simulink model "blockdemo_accumulationchaining"  (Simulink 7.6)
settings: Solver=ode45  StartTime=0.0  StopTime=10.0  RelTol=1e-3
InitFcn:
  | %% DSPBuilder Start
  | alt_dspbuilder_update_model(bdroot)
  | %% DSPBuilder End
libraries: allblocks_alteradspbuilder2 x14, simulink x2
settings Model: Creator=akarapet  LastModifiedBy=akarapet

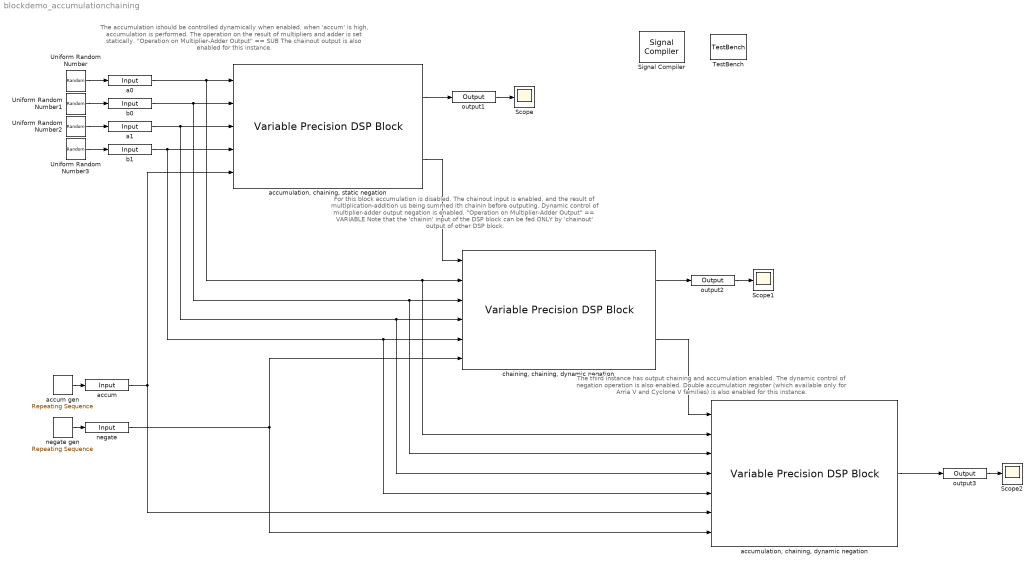
== system blockdemo_accumulationchaining ==
  note: The accumulation ishould be controlled dynamically when enabled.
      | when 'accum' is high, accumulation is performed.
      | The operation on the result of multipliers and adder is set statically.
      | "Operation on Multiplier-Adder Output" == SUB
      | The chainout output is also enabled for this instance.
  note: For this block accumulation is disabled.
      | The chainout input is enabled, and the result of multiplication-addition
      | us being summed ith chainin before outputing.
      | Dynamic control of multiplier-adder output negation is enabled.
      | "Operation on Multiplier-Adder Output" == VARIABLE
      |
      | Note that the 'chainin' input of the DSP block can be fed ONLY
      | by 'chainout' output of other DSP block.
  note: The third instance has output chaining and accumulation enabled.
      | The dynamic control of negation operation is also enabled.
      | Double accumulation register (which available only for Arria V and
      | Cyclone V families) is also enabled for this instance.
  Scope : Scope
  Scope1 : Scope
  Scope2 : Scope
      settings: SaveName=ScopeData2
  Signal Compiler : allblocks_alteradspbuilder2/Signal Compiler  DeviceFamily=Arria V  DeviceName=AUTO  EnableSignalTap=off  SignalTapDepth=128  UseBoardBlock=off  StpUseDefaultClock=on  StpClock=Clock  ExportDir=/data/akarapet/qshell_linux64_regtests/p4/regtest/ip/dspb/basiclibrarytests/arithmetic/stratixvdsp/basicchainaccum
  TestBench : allblocks_alteradspbuilder2/TestBench  enable=on  advancedMode=off  modelSimGui=off  maxDisplayErrors=10  mismatchErrorLevel=Error  simdatafile=/data/akarapet/qshell_linux64_regtests/p4/dsp_builder/dsp_builder2/Documentation/DesignExamples/Tutorials/UnitBlocks/Arithmetic/VariablePrecisionDSPBlock/tb_blockdemo_accumulationchaining/blockdemo_accumulationchaining.simdata.tcl
  Uniform Random Number : UniformRandomNumber  Minimum=-128  Maximum=128  Seed=1231  SampleTime=1
  Uniform Random Number1 : UniformRandomNumber  Minimum=-128  Maximum=128  Seed=2365  SampleTime=1
  Uniform Random Number2 : UniformRandomNumber  Minimum=-128  Maximum=128  Seed=1234  SampleTime=1
  Uniform Random Number3 : UniformRandomNumber  Minimum=-128  Maximum=128  Seed=2365  SampleTime=1
  a0 : allblocks_alteradspbuilder2/Input  iofile=/data/akarapet/qshell_linux64_regtests/p4/dsp_builder/dsp_builder2/Documentation/DesignExamples/Tutorials/UnitBlocks/Arithmetic/VariablePrecisionDSPBlock/tb_blockdemo_accumulationchaining/blockdemo%5Faccumulationchaining_a0.salt  BusType=Signed Integer  bwl=8  bwr=0  SpecifyClock=off  clock=default_clock  PORTTYPE=Input  externalType=Inferred  allowFloatingPointOverride=on  logOutputs=off
  a1 : allblocks_alteradspbuilder2/Input  iofile=/data/akarapet/qshell_linux64_regtests/p4/dsp_builder/dsp_builder2/Documentation/DesignExamples/Tutorials/UnitBlocks/Arithmetic/VariablePrecisionDSPBlock/tb_blockdemo_accumulationchaining/blockdemo%5Faccumulationchaining_a1.salt  BusType=Signed Integer  bwl=8  bwr=0  SpecifyClock=off  clock=default_clock  PORTTYPE=Input  externalType=Inferred  allowFloatingPointOverride=on  logOutputs=off
  accum : allblocks_alteradspbuilder2/Input  iofile=/data/akarapet/qshell_linux64_regtests/p4/dsp_builder/dsp_builder2/Documentation/DesignExamples/Tutorials/UnitBlocks/Arithmetic/VariablePrecisionDSPBlock/tb_blockdemo_accumulationchaining/blockdemo%5Faccumulationchaining_accum.salt  BusType=Single Bit  bwl=8  bwr=0  SpecifyClock=off  clock=default_clock  PORTTYPE=Input  externalType=Inferred  allowFloatingPointOverride=on  logOutputs=off
  accum gen : simulink/Sources/Repeating Sequence  SystemSampleTime=-1  rep_seq_t=[0 1 2 3 4 5 6 7]  rep_seq_y=[1 1 1 0 0 0 1 1]
  "accumulation, chaining, dynamic negation" : allblocks_alteradspbuilder2/Variable Precision DSP Block  complex_model_delayed=0  model_delayed=0  device_family=Arria V  used_mode_stratix=Other Modes  used_mode_arria=Other Modes  in_25x18_complex_mode=0  in_18x18plus36_mode=0  in_other_modes=1  number_of_mults=2  clock_ena_inputs=off  async_clear_inputs=off  bus_type=Signed Integer  bwl_A=8  bwr_A=0  width_A=8  chain_width=64  reg_inputs_A=off  A_inputs_reg_ena=ENABLE 0  bwl_B=8  bwr_B=0  width_B=8  reg_inputs_B=on  B_inputs_reg_ena=ENABLE 0  bwl_joint_A_B=8  bwr_joint_A_B=0  reg_joint_A_B_input=on  A_B_input_reg_ena=ENABLE 0  bwl_A_complex=8  bwr_A_complex=8  reg_complex_A=on  A_complex_inputs_reg_ena=ENABLE 0  bwl_B_complex=8  bwr_B_complex=8  reg_complex_B=on  B_complex_inputs_reg_ena=ENABLE 0  A_inputs_exist=1  B_inputs_exist=1  C_inputs_exist=0  coef_sel_inputs_exist=0  all_inputs_registered=0  no_input_registered=0  all_inputs_share_same_clocks=0  full_resolution=off  bwl_out=32  bwr_out=0  reg_output=on  output_reg_ena=ENABLE 0  systolic_regs_available=1  enable_systolic_regs=off  systolic_regs_used=0  basic_struct_ok_for_input_scan=1  input_scan_available=0  enable_input_scan=off  input_scan_used=0  input_scan_delay_regs_available=0  enable_input_scan_delay_regs=off  input_scan_delay_regs_used=0  basic_struct_ok_for_coef_rom=1  coef_rom_available=0  enable_coef_rom=off  coef_rom_used=0  basic_struct_ok_for_preadder=1  preadder_available=0  enable_preadder=off  preadder_used=0  preadder_direction=ADD  square_mode_available=0  enable_square_mode=off  square_mode_used=0  upper_limit_9bit=9  upper_limit_18bit=19  upper_limit_27bit=27  in_18x18_modes=1  in_27x27_modes=0  in_36x18_modes=0  in_36x36_mode=0  mult1_adder_available=1  mult1_direction=ADD  mult3_adder_available=0  mult3_direction=ADD  chainout_adder_available=1  use_chainout_input=on  chainout_input_used=1  use_chainout_output=off  chainout_output_used=0  accum_available=1  enable_accum=on  accum_used=1  double_accum_available=1  enable_double_accum=on  double_accum_used=1  negate_available=1  mult_add_operation=VARIABLE  rounding_constant_available=1  use_rounding_constant=off  rounding_constant_used=0  constant_value=1  bwl_C=8  bwr_C=0  bwl_coef=18  bwr_coef=0  mult0_coeffs=[0, 0, 0, 0, 0, 0, 0, 0]  mult1_coeffs=[0, 0, 0, 0, 0, 0, 0, 0]  mult2_coeffs=[0, 0, 0, 0, 0, 0, 0, 0]  mult3_coeffs=[0, 0, 0, 0, 0, 0, 0, 0]  reg_mult1_op_control=off  reg_mult3_op_control=off  reg_accum_control=off  reg_negate_control=off  control_regs_ena=ENABLE 0
  "accumulation, chaining, static negation" : allblocks_alteradspbuilder2/Variable Precision DSP Block  complex_model_delayed=0  model_delayed=0  device_family=Arria V  used_mode_stratix=Other Modes  used_mode_arria=Other Modes  in_25x18_complex_mode=0  in_18x18plus36_mode=0  in_other_modes=1  number_of_mults=2  clock_ena_inputs=off  async_clear_inputs=off  bus_type=Signed Integer  bwl_A=8  bwr_A=0  width_A=8  chain_width=64  reg_inputs_A=on  A_inputs_reg_ena=ENABLE 0  bwl_B=8  bwr_B=0  width_B=8  reg_inputs_B=off  B_inputs_reg_ena=ENABLE 0  bwl_joint_A_B=8  bwr_joint_A_B=0  reg_joint_A_B_input=on  A_B_input_reg_ena=ENABLE 0  bwl_A_complex=8  bwr_A_complex=8  reg_complex_A=on  A_complex_inputs_reg_ena=ENABLE 0  bwl_B_complex=8  bwr_B_complex=8  reg_complex_B=on  B_complex_inputs_reg_ena=ENABLE 0  A_inputs_exist=1  B_inputs_exist=1  C_inputs_exist=0  coef_sel_inputs_exist=0  all_inputs_registered=0  no_input_registered=0  all_inputs_share_same_clocks=0  full_resolution=off  bwl_out=32  bwr_out=0  reg_output=on  output_reg_ena=ENABLE 0  systolic_regs_available=1  enable_systolic_regs=off  systolic_regs_used=0  basic_struct_ok_for_input_scan=1  input_scan_available=0  enable_input_scan=off  input_scan_used=0  input_scan_delay_regs_available=0  enable_input_scan_delay_regs=off  input_scan_delay_regs_used=0  basic_struct_ok_for_coef_rom=1  coef_rom_available=0  enable_coef_rom=off  coef_rom_used=0  basic_struct_ok_for_preadder=1  preadder_available=0  enable_preadder=off  preadder_used=0  preadder_direction=ADD  square_mode_available=0  enable_square_mode=off  square_mode_used=0  upper_limit_9bit=9  upper_limit_18bit=19  upper_limit_27bit=27  in_18x18_modes=1  in_27x27_modes=0  in_36x18_modes=0  in_36x36_mode=0  mult1_adder_available=1  mult1_direction=SUB  mult3_adder_available=0  mult3_direction=ADD  chainout_adder_available=1  use_chainout_input=off  chainout_input_used=0  use_chainout_output=on  chainout_output_used=1  accum_available=1  enable_accum=on  accum_used=1  double_accum_available=1  enable_double_accum=off  double_accum_used=0  negate_available=1  mult_add_operation=SUB  rounding_constant_available=1  use_rounding_constant=off  rounding_constant_used=0  constant_value=1  bwl_C=8  bwr_C=0  bwl_coef=18  bwr_coef=0  mult0_coeffs=[0, 0, 0, 0, 0, 0, 0, 0]  mult1_coeffs=[0, 0, 0, 0, 0, 0, 0, 0]  mult2_coeffs=[0, 0, 0, 0, 0, 0, 0, 0]  mult3_coeffs=[0, 0, 0, 0, 0, 0, 0, 0]  reg_mult1_op_control=off  reg_mult3_op_control=off  reg_accum_control=off  reg_negate_control=off  control_regs_ena=ENABLE 0
  b0 : allblocks_alteradspbuilder2/Input  iofile=/data/akarapet/qshell_linux64_regtests/p4/dsp_builder/dsp_builder2/Documentation/DesignExamples/Tutorials/UnitBlocks/Arithmetic/VariablePrecisionDSPBlock/tb_blockdemo_accumulationchaining/blockdemo%5Faccumulationchaining_b0.salt  BusType=Signed Integer  bwl=8  bwr=0  SpecifyClock=off  clock=default_clock  PORTTYPE=Input  externalType=Inferred  allowFloatingPointOverride=on  logOutputs=off
  b1 : allblocks_alteradspbuilder2/Input  iofile=/data/akarapet/qshell_linux64_regtests/p4/dsp_builder/dsp_builder2/Documentation/DesignExamples/Tutorials/UnitBlocks/Arithmetic/VariablePrecisionDSPBlock/tb_blockdemo_accumulationchaining/blockdemo%5Faccumulationchaining_b1.salt  BusType=Signed Integer  bwl=8  bwr=0  SpecifyClock=off  clock=default_clock  PORTTYPE=Input  externalType=Inferred  allowFloatingPointOverride=on  logOutputs=off
  "chaining, chaining, dynamic negation" : allblocks_alteradspbuilder2/Variable Precision DSP Block  complex_model_delayed=0  model_delayed=0  device_family=Arria V  used_mode_stratix=Other Modes  used_mode_arria=Other Modes  in_25x18_complex_mode=0  in_18x18plus36_mode=0  in_other_modes=1  number_of_mults=2  clock_ena_inputs=off  async_clear_inputs=off  bus_type=Signed Integer  bwl_A=8  bwr_A=0  width_A=8  chain_width=64  reg_inputs_A=off  A_inputs_reg_ena=ENABLE 0  bwl_B=8  bwr_B=0  width_B=8  reg_inputs_B=off  B_inputs_reg_ena=ENABLE 0  bwl_joint_A_B=8  bwr_joint_A_B=0  reg_joint_A_B_input=on  A_B_input_reg_ena=ENABLE 0  bwl_A_complex=8  bwr_A_complex=8  reg_complex_A=on  A_complex_inputs_reg_ena=ENABLE 0  bwl_B_complex=8  bwr_B_complex=8  reg_complex_B=on  B_complex_inputs_reg_ena=ENABLE 0  A_inputs_exist=1  B_inputs_exist=1  C_inputs_exist=0  coef_sel_inputs_exist=0  all_inputs_registered=0  no_input_registered=1  all_inputs_share_same_clocks=1  full_resolution=off  bwl_out=32  bwr_out=0  reg_output=on  output_reg_ena=ENABLE 0  systolic_regs_available=1  enable_systolic_regs=off  systolic_regs_used=0  basic_struct_ok_for_input_scan=1  input_scan_available=0  enable_input_scan=off  input_scan_used=0  input_scan_delay_regs_available=0  enable_input_scan_delay_regs=off  input_scan_delay_regs_used=0  basic_struct_ok_for_coef_rom=1  coef_rom_available=1  enable_coef_rom=off  coef_rom_used=0  basic_struct_ok_for_preadder=1  preadder_available=1  enable_preadder=off  preadder_used=0  preadder_direction=ADD  square_mode_available=0  enable_square_mode=off  square_mode_used=0  upper_limit_9bit=9  upper_limit_18bit=19  upper_limit_27bit=27  in_18x18_modes=1  in_27x27_modes=0  in_36x18_modes=0  in_36x36_mode=0  mult1_adder_available=1  mult1_direction=ADD  mult3_adder_available=0  mult3_direction=ADD  chainout_adder_available=1  use_chainout_input=on  chainout_input_used=1  use_chainout_output=on  chainout_output_used=1  accum_available=1  enable_accum=off  accum_used=0  double_accum_available=0  enable_double_accum=off  double_accum_used=0  negate_available=1  mult_add_operation=VARIABLE  rounding_constant_available=1  use_rounding_constant=off  rounding_constant_used=0  constant_value=1  bwl_C=8  bwr_C=0  bwl_coef=18  bwr_coef=0  mult0_coeffs=[0, 0, 0, 0, 0, 0, 0, 0]  mult1_coeffs=[0, 0, 0, 0, 0, 0, 0, 0]  mult2_coeffs=[0, 0, 0, 0, 0, 0, 0, 0]  mult3_coeffs=[0, 0, 0, 0, 0, 0, 0, 0]  reg_mult1_op_control=off  reg_mult3_op_control=off  reg_accum_control=off  reg_negate_control=on  control_regs_ena=ENABLE 0
  negate : allblocks_alteradspbuilder2/Input  iofile=/data/akarapet/qshell_linux64_regtests/p4/dsp_builder/dsp_builder2/Documentation/DesignExamples/Tutorials/UnitBlocks/Arithmetic/VariablePrecisionDSPBlock/tb_blockdemo_accumulationchaining/blockdemo%5Faccumulationchaining_negate.salt  BusType=Single Bit  bwl=8  bwr=0  SpecifyClock=off  clock=default_clock  PORTTYPE=Input  externalType=Inferred  allowFloatingPointOverride=on  logOutputs=off
  negate gen : simulink/Sources/Repeating Sequence  SystemSampleTime=-1  rep_seq_t=[0 1 2 3 4 5 6 7]  rep_seq_y=[1 0 1 0 0 1 1 1]
  output1 : allblocks_alteradspbuilder2/Output  iofile=/data/akarapet/qshell_linux64_regtests/p4/dsp_builder/dsp_builder2/Documentation/DesignExamples/Tutorials/UnitBlocks/Arithmetic/VariablePrecisionDSPBlock/tb_blockdemo_accumulationchaining/blockdemo%5Faccumulationchaining_output1.capture  BusType=Signed Integer  bwl=32  bwr=0  externalType=Inferred  PORTTYPE=Output  allowFloatingPointOverride=on  logOutputs=off
  output2 : allblocks_alteradspbuilder2/Output  iofile=/data/akarapet/qshell_linux64_regtests/p4/dsp_builder/dsp_builder2/Documentation/DesignExamples/Tutorials/UnitBlocks/Arithmetic/VariablePrecisionDSPBlock/tb_blockdemo_accumulationchaining/blockdemo%5Faccumulationchaining_output2.capture  BusType=Signed Integer  bwl=32  bwr=0  externalType=Inferred  PORTTYPE=Output  allowFloatingPointOverride=on  logOutputs=off
  output3 : allblocks_alteradspbuilder2/Output  iofile=/data/akarapet/qshell_linux64_regtests/p4/dsp_builder/dsp_builder2/Documentation/DesignExamples/Tutorials/UnitBlocks/Arithmetic/VariablePrecisionDSPBlock/tb_blockdemo_accumulationchaining/blockdemo%5Faccumulationchaining_output3.capture  BusType=Signed Integer  bwl=32  bwr=0  externalType=Inferred  PORTTYPE=Output  allowFloatingPointOverride=on  logOutputs=off
  wires:
  Uniform Random Number/1 -> a0/1
  Uniform Random Number1/1 -> b0/1
  "accumulation, chaining, static negation"/1 -> output1/1
  Uniform Random Number2/1 -> a1/1
  Uniform Random Number3/1 -> b1/1
  "accumulation, chaining, dynamic negation"/1 -> output3/1
  a0/1 -> "accumulation, chaining, static negation"/1, "chaining, chaining, dynamic negation"/2, "accumulation, chaining, dynamic negation"/2
  b0/1 -> "accumulation, chaining, static negation"/2, "chaining, chaining, dynamic negation"/3, "accumulation, chaining, dynamic negation"/3
  a1/1 -> "accumulation, chaining, static negation"/3, "chaining, chaining, dynamic negation"/4, "accumulation, chaining, dynamic negation"/4
  b1/1 -> "accumulation, chaining, static negation"/4, "chaining, chaining, dynamic negation"/5, "accumulation, chaining, dynamic negation"/5
  accum gen/1 -> accum/1
  negate gen/1 -> negate/1
  "accumulation, chaining, static negation"/2 -> "chaining, chaining, dynamic negation"/1
  "chaining, chaining, dynamic negation"/1 -> output2/1
  "chaining, chaining, dynamic negation"/2 -> "accumulation, chaining, dynamic negation"/1
  accum/1 -> "accumulation, chaining, static negation"/5, "accumulation, chaining, dynamic negation"/6
  negate/1 -> "chaining, chaining, dynamic negation"/6, "accumulation, chaining, dynamic negation"/7
  output1/1 -> Scope/1
  output2/1 -> Scope1/1
  output3/1 -> Scope2/1
